simulink model "W1985546_20222145_Model_system"  (R2023b)
settings: Solver=VariableStepAuto  StartTime=0.0  StopTime=10.0  RelTol=1e-3
settings Model: Creator=Acer  LastModifiedBy=Acer

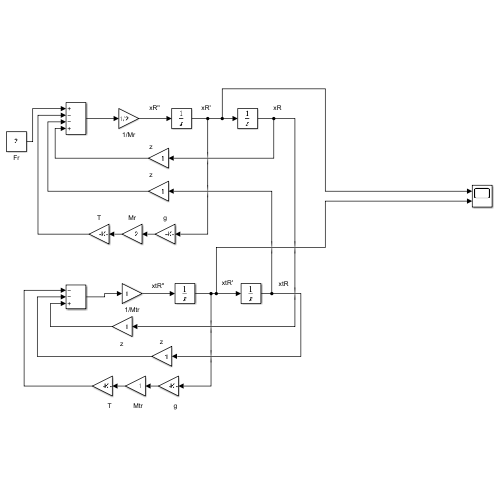
[thumbnail: Simulink's stored preview of the top-level diagram]
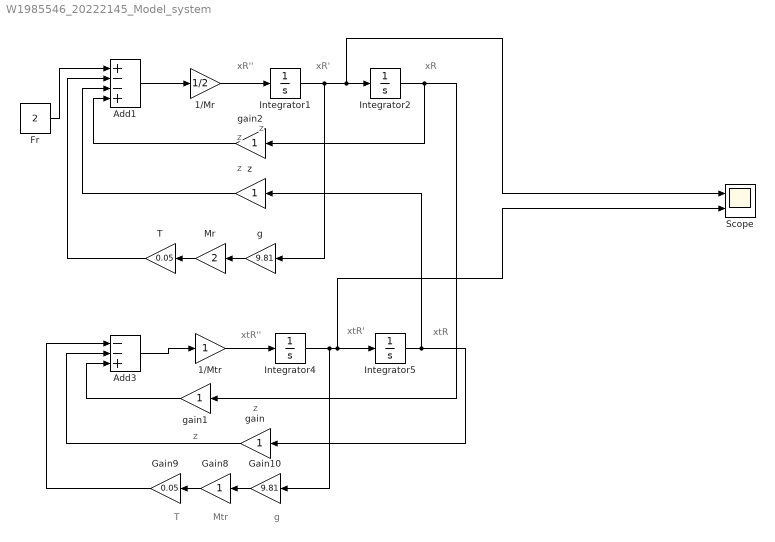
== system W1985546_20222145_Model_system ==
  note: z
  note: xtR
  note: z
  note: z
  note: xR'
  note: xtR''
  note: g
  note: z
  note: z
  note: Mtr
  note: xtR'
  note: xR''
  note: T
  note: xR
  1/Mr : Gain  Gain=1/2
  1/Mtr : Gain
  Add1 : Sum  Inputs=+--+
  Add3 : Sum  Inputs=--+
  Fr : Constant  Value=2
  Gain10 : Gain  Gain=9.81
  Gain8 : Gain
  Gain9 : Gain  Gain=0.05
  Integrator{1..2,4..5} (4 alike) : Integrator
  Mr : Gain  Gain=2
  Scope : Scope  NumInputPorts=2
  T : Gain  Gain=0.05
  g : Gain  Gain=9.81
  gain : Gain
  gain1 : Gain
  gain2 : Gain
  z : Gain
  wires:
  gain2/1 -> Add1/4
  gain/1 -> Add3/2
  Mr/1 -> T/1
  z/1 -> Add1/3
  Gain9/1 -> Add3/1
  Gain8/1 -> Gain9/1
  Integrator4/1 -> Integrator5/1, Scope/2, Gain10/1
  Add1/1 -> 1/Mr/1
  Gain10/1 -> Gain8/1
  Integrator1/1 -> Scope/1, Integrator2/1, g/1
  T/1 -> Add1/2
  gain1/1 -> Add3/3
  1/Mtr/1 -> Integrator4/1
  1/Mr/1 -> Integrator1/1
  Integrator2/1 -> gain1/1, gain2/1
  Fr/1 -> Add1/1
  Add3/1 -> 1/Mtr/1
  Integrator5/1 -> gain/1, z/1
  g/1 -> Mr/1
